simulink model "Evita_Paredes_Sist_Completo"  (R2023b)
settings: Solver=FixedStepAuto  StartTime=0.0  StopTime=inf  RelTol=1e-3  EnableMultiTasking=on
libraries: simulink x7
settings Model: ExtModeTrigDuration=2  Creator=marqu  LastModifiedBy=marqu
settings SolverCC: AutoInsertRateTranBlk=on
settings OptimizationCC: EnhancedBackFolding=on  PassReuseOutputArgsAs=Individual arguments  ZeroExternalMemoryAtStartup=off  ZeroInternalMemoryAtStartup=off  MaxStackSize=64  OptimizeBlockOrder=speed  DifferentSizesBufferReuse=on  OptimizationCustomize=off  EfficientTunableParamExpr=on
settings DebuggingCC: ParameterTunabilityLossMsg=error
settings HardwareCC: ProdBitPerInt=16  ProdBitPerPointer=16  ProdBitPerSizeT=16  ProdBitPerPtrDiffT=16  ProdLargestAtomicFloat=None  ProdWordSize=8  ProdHWDeviceType=Atmel->AVR
settings SFSimCC: MATLABDynamicMemAlloc=off
settings RTWCC: Description=Embedded Coder  SystemTargetFile=ert.tlc  HardwareBoard=Arduino Mega 2560  TemplateMakefile=ert_default_tmf  Toolchain=Arduino AVR  BuildConfiguration=Faster Runs
settings CodeAppCC: ForceParamTrailComments=on  IgnoreCustomStorageClasses=off  OperatorAnnotations=on  SimulinkDataObjDesc=on  SFDataObjDesc=on  InsertBlockDesc=on
settings ERTTargetCC: SupportContinuousTime=on  SupportVariableSizeSignals=on  ExtModeTransport=3  ExtModeStaticAlloc=on  ExtModeAutomaticAllocSize=off  ExtModeStaticAllocSize=2048  ExtModeMexFile=ext_xcp  ExtModeIntrfLevel=Level2 - Open

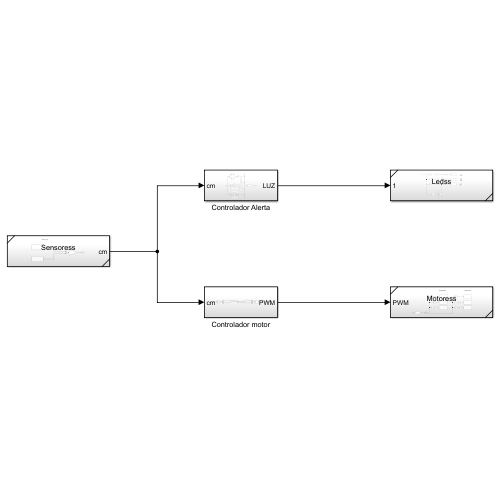
[thumbnail: Simulink's stored preview of the top-level diagram]
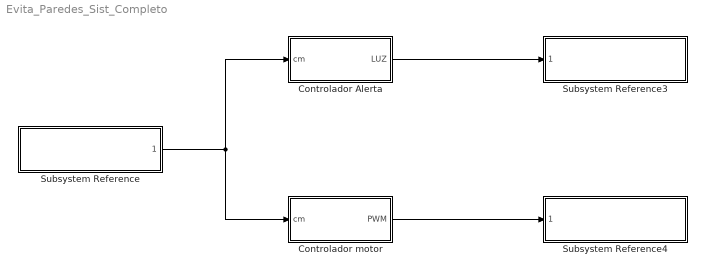
== system Evita_Paredes_Sist_Completo ==
  Controlador Alerta : Subsystem
  Controlador motor : Subsystem
  Subsystem Reference : Subsystem  ReferencedSubsystem=Sensoress
  Subsystem Reference3 : Subsystem  ReferencedSubsystem=Ledss
  Subsystem Reference4 : Subsystem  ReferencedSubsystem=Motoress
  wires:
  Subsystem Reference/1 -> Controlador motor/1(cm), Controlador Alerta/1(cm)
  Controlador Alerta/1(LUZ) -> Subsystem Reference3/1
  Controlador motor/1(PWM) -> Subsystem Reference4/1

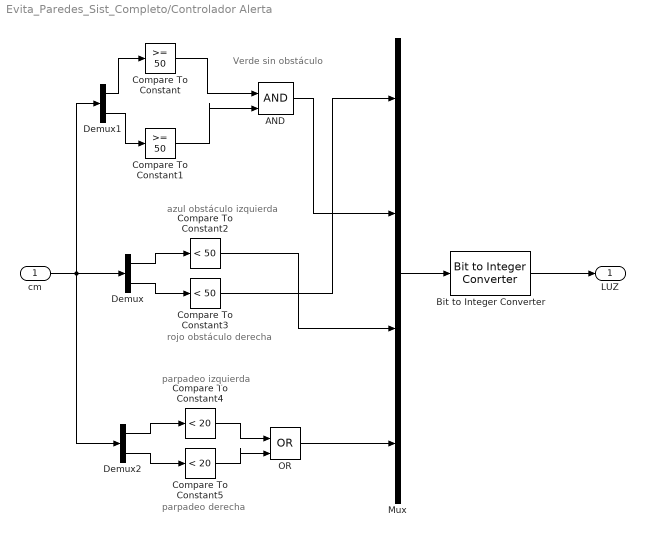
== system Evita_Paredes_Sist_Completo/Controlador Alerta ==
  note: azul obstáculo izquierda
  note: Verde sin obstáculo
  note: rojo obstáculo derecha
  note: parpadeo izquierda
  note: parpadeo derecha
  cm : Inport
  AND : Logic  IconShape=distinctive  AllPortsSameDT=off  OutDataTypeStr=boolean
  Bit to Integer Converter : simulink/Logic and Bit Operations/Bit to Integer Converter  nbits=4  bitOrder=MSB first  signedOutputValues=Unsigned  outDtype=uint8  outDtypeSigned=Inherit via internal rule
      settings: LibrarySourceBlock=|
      | commutil2/Bit to Integer
      | Converter
  Compare To Constant : simulink/Logic and Bit Operations/Compare To Constant  relop=>=  const=50  OutDataTypeStr=boolean
  Compare To Constant1 : simulink/Logic and Bit Operations/Compare To Constant  relop=>=  const=50  OutDataTypeStr=boolean
  Compare To Constant2 : simulink/Logic and Bit Operations/Compare To Constant  relop=<  const=50  OutDataTypeStr=boolean
  Compare To Constant3 : simulink/Logic and Bit Operations/Compare To Constant  relop=<  const=50  OutDataTypeStr=boolean
  Compare To Constant4 : simulink/Logic and Bit Operations/Compare To Constant  relop=<  const=20  OutDataTypeStr=boolean
  Compare To Constant5 : simulink/Logic and Bit Operations/Compare To Constant  relop=<  const=20  OutDataTypeStr=boolean
  Demux : Demux  Outputs=2
  Demux1 : Demux  Outputs=2
  Demux2 : Demux  Outputs=2
  Mux : Mux
  OR : Logic  Operator=OR  IconShape=distinctive  AllPortsSameDT=off  OutDataTypeStr=boolean
  LUZ : Outport
  wires:
  cm/1 -> Demux2/1, Demux1/1, Demux/1
  Compare To Constant/1 -> AND/1
  Compare To Constant1/1 -> AND/2
  Demux1/1 -> Compare To Constant/1
  Demux1/2 -> Compare To Constant1/1
  Demux/1 -> Compare To Constant2/1
  Demux/2 -> Compare To Constant3/1
  Demux2/1 -> Compare To Constant4/1
  Demux2/2 -> Compare To Constant5/1
  Compare To Constant4/1 -> OR/1
  Compare To Constant5/1 -> OR/2
  Bit to Integer Converter/1 -> LUZ/1
  OR/1 -> Mux/4
  Mux/1 -> Bit to Integer Converter/1
  Compare To Constant3/1 -> Mux/1
  AND/1 -> Mux/2
  Compare To Constant2/1 -> Mux/3

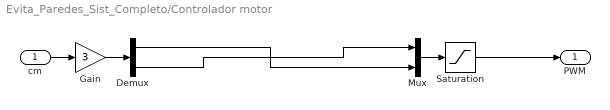
== system Evita_Paredes_Sist_Completo/Controlador motor ==
  cm : Inport
  Demux : Demux  Outputs=2
  Gain : Gain  Gain=3
  Mux : Mux  Inputs=2
  Saturation : Saturate  UpperLimit=80  LowerLimit=0  OutDataTypeStr=int16
  PWM : Outport
  wires:
  Gain/1 -> Demux/1
  cm/1 -> Gain/1
  Mux/1 -> Saturation/1
  Saturation/1 -> PWM/1
  Demux/1 -> Mux/2
  Demux/2 -> Mux/1
